simulink model "ExtINS_DataSIM"  (R2018b)
settings: Solver=FixedStepDiscrete  StartTime=start_time  StopTime=INS_Out.timestamp.Time(end)  FixedStep=0.001  RelTol=1e-3
InitFcn:
  | load_parameter
  | mission_data_preprocess
settings Model: Creator=zouj  LastModifiedBy=zouji
settings OptimizationCC: DefaultUnderspecifiedDataType=single  EfficientMapNaN2IntZero=off
settings DebuggingCC: ParameterOverflowMsg=none  UnconnectedInputMsg=none  UnconnectedOutputMsg=none  UnconnectedLineMsg=none
settings HardwareCC: TargetBitPerPointer=64  TargetBitPerSizeT=64  TargetBitPerPtrDiffT=64  TargetLongLongMode=on  TargetIntDivRoundTo=Zero  TargetEndianess=LittleEndian  TargetWordSize=64  TargetHWDeviceType=MATLAB Host  ProdEqTarget=off
settings ModelReferenceCC: ModelReferenceNumInstancesAllowed=Single
settings CodeAppCC: MaxIdLength=128
settings GRTTargetCC: TargetLangStandard=C89/C90 (ANSI)  CombineOutputUpdateFcns=off  GRTInterface=on

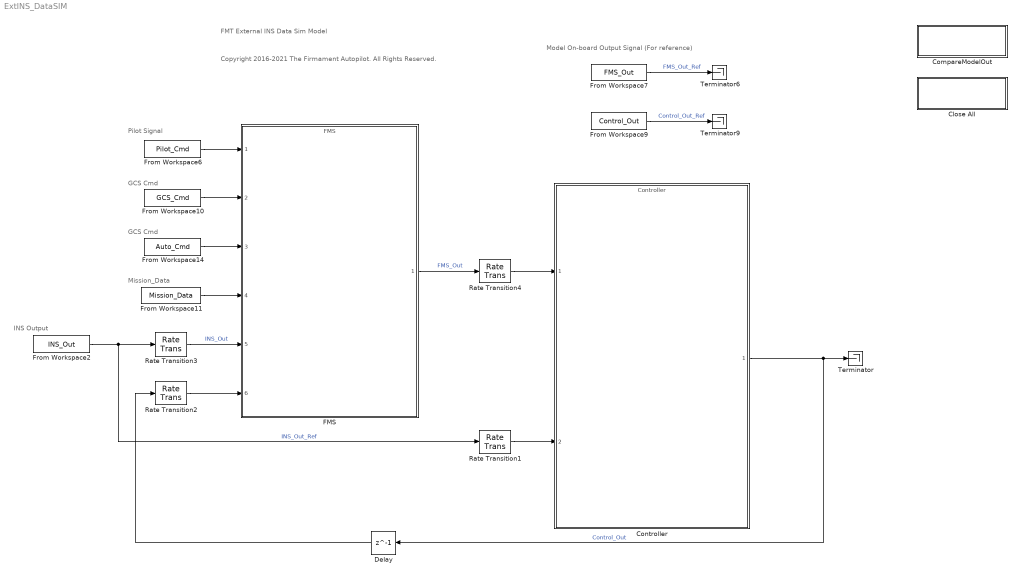
== system ExtINS_DataSIM ==
  note: Pilot Signal
  note: Model On-board Output Signal (For reference)
  note: FMT External INS Data Sim Model
  note: Copyright 2016-2021 The Firmament Autopilot. All Rights Reserved.
  note: GCS Cmd
  note: Mission_Data
  note: GCS Cmd
  note: INS Output
  Close All : Subsystem
      settings: OpenFcn=close all;
  CompareModelOut : Subsystem
      settings: OpenFcn=compareModelOut;
  Controller : ModelReference  ModelNameDialog=Controller.slx  ModelReferenceVersion=1.1023
  Delay : Delay  DelayLength=1
  FMS : ModelReference  ModelNameDialog=FMS.slx  ModelReferenceVersion=1.2335
  From Workspace10 : FromWorkspace  VariableName=GCS_Cmd  OutDataTypeStr=Bus: GCS_Cmd_Bus  Interpolate=off  OutputAfterFinalValue=Holding final value
  From Workspace11 : FromWorkspace  VariableName=Mission_Data  OutDataTypeStr=Bus: Mission_Data_Bus  Interpolate=off  OutputAfterFinalValue=Holding final value
  From Workspace14 : FromWorkspace  VariableName=Auto_Cmd  OutDataTypeStr=Bus: Auto_Cmd_Bus  Interpolate=off  OutputAfterFinalValue=Holding final value
  From Workspace2 : FromWorkspace  VariableName=INS_Out  OutDataTypeStr=Bus: INS_Out_Bus  Interpolate=off  OutputAfterFinalValue=Holding final value
  From Workspace6 : FromWorkspace  VariableName=Pilot_Cmd  OutDataTypeStr=Bus: Pilot_Cmd_Bus  Interpolate=off  OutputAfterFinalValue=Holding final value
  From Workspace7 : FromWorkspace  VariableName=FMS_Out  OutDataTypeStr=Bus: FMS_Out_Bus  Interpolate=off  OutputAfterFinalValue=Holding final value
  From Workspace9 : FromWorkspace  VariableName=Control_Out  OutDataTypeStr=Bus: Control_Out_Bus  Interpolate=off  OutputAfterFinalValue=Holding final value
  Rate Transition1 : RateTransition  OutPortSampleTime=CONTROL_CONST.dt
  Rate Transition2 : RateTransition  OutPortSampleTime=FMS_CONST.dt
  Rate Transition3 : RateTransition  OutPortSampleTime=FMS_CONST.dt
  Rate Transition4 : RateTransition  OutPortSampleTime=CONTROL_CONST.dt
  Terminator : Terminator
  Terminator6 : Terminator
  Terminator9 : Terminator
  wires:
  Rate Transition1/1 -> Controller/2
  From Workspace2/1 -> Rate Transition3/1, Rate Transition1/1  "INS_Out_Ref"
  FMS/1 -> Rate Transition4/1  "FMS_Out"
  From Workspace6/1 -> FMS/1
  Controller/1 -> Delay/1, Terminator/1  "Control_Out"
  From Workspace7/1 -> Terminator6/1  "FMS_Out_Ref"
  From Workspace9/1 -> Terminator9/1  "Control_Out_Ref"
  Delay/1 -> Rate Transition2/1
  Rate Transition4/1 -> Controller/1
  Rate Transition2/1 -> FMS/6
  Rate Transition3/1 -> FMS/5  "INS_Out"
  From Workspace10/1 -> FMS/2
  From Workspace14/1 -> FMS/3
  From Workspace11/1 -> FMS/4

== system ExtINS_DataSIM/Close All ==

== system ExtINS_DataSIM/CompareModelOut ==
